simulink model "tension_inverter_2016"  (R2016b)
settings: Solver=FixedStepAuto  StartTime=0.0  StopTime=t_max  FixedStep=timestep  RelTol=1e-3
values from neighbouring files (symbols this model uses):
  Cf = 50e-6    (= 5e-05)    [script.m]
  K = (Lf*Rg)/Lg    (= 1.33333333333)    [script.m]
  Lf = 1e-3    (= 0.001)    [script.m]
  Lg = 150e-6    (= 0.00015)    [script.m]
  Rg = 0.2    [script.m]
  step_v = 1    [script.m]
settings Model: Creator=mluser  LastModifiedBy=Gabriel
settings DataIOCC: ReturnWorkspaceOutputs=on
settings DebuggingCC: UnconnectedInputMsg=none  UnconnectedOutputMsg=none  UnconnectedLineMsg=none
settings ModelReferenceCC: EnableRefExpFcnMdlSchedulingChecks=off
settings SFSimCC: SimUseLocalCustomCode=on
settings RTWCC: RTWUseLocalCustomCode=on

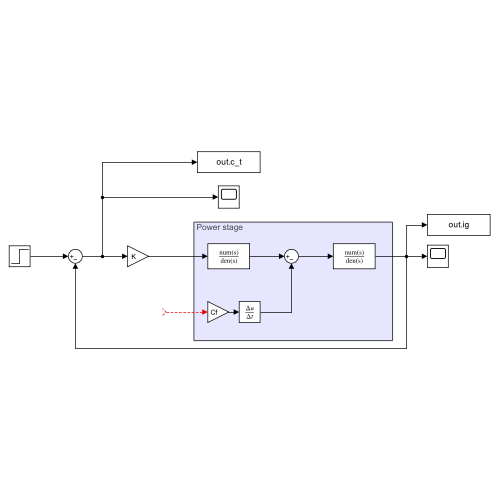
[thumbnail: Simulink's stored preview of the top-level diagram]
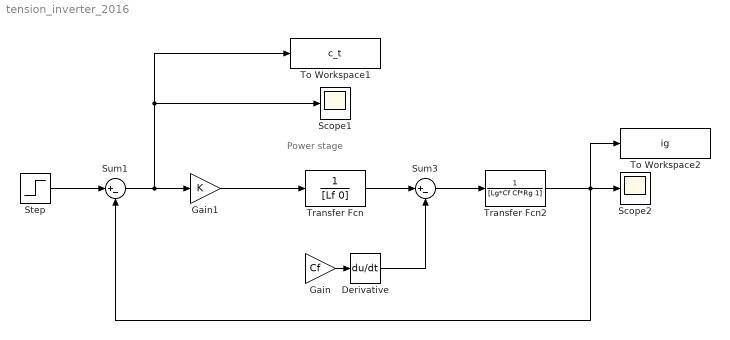
== system tension_inverter_2016 ==
  note: Power stage
  Derivative : Derivative
  Gain : Gain  Gain=Cf
  Gain1 : Gain  Gain=K
  Scope1 : Scope
  Scope2 : Scope
  Step : Step  Time=0  After=step_v  SampleTime=0
  Sum1 : Sum  Inputs=|+-
  Sum3 : Sum  Inputs=|+-
  To Workspace1 : ToWorkspace  VariableName=c_t  SampleTime=-1
  To Workspace2 : ToWorkspace  VariableName=ig  SampleTime=-1
  Transfer Fcn : TransferFcn  Denominator=[Lf 0]
  Transfer Fcn2 : TransferFcn  Denominator=[Lg*Cf Cf*Rg 1]
  wires:
  Transfer Fcn/1 -> Sum3/1
  ? -> Gain/1
  Sum3/1 -> Transfer Fcn2/1
  Transfer Fcn2/1 -> To Workspace2/1, Scope2/1, Sum1/2
  Step/1 -> Sum1/1
  Sum1/1 -> Gain1/1, Scope1/1, To Workspace1/1
  Gain/1 -> Derivative/1
  Derivative/1 -> Sum3/2
  Gain1/1 -> Transfer Fcn/1
